simulink model "Copy_2_of_Constant_vel"  (R2024b)
settings: Solver=FixedStepAuto  StartTime=0.0  StopTime=10  FixedStep=0.001  RelTol=1e-3
values from neighbouring files (symbols this model uses):
  marker_data = [marker_data, [20;80;0.5]]    [setup.m]
undefined symbols (not defined in the file or in its folder): r_a, r_b, r_c
libraries: simulink x5, aerolibutil x1, shared6dof x1, aerolibanim x1, aerolibnav x1
(part 2 of 2)

== matlab function Copy_2_of_Constant_vel/MATLAB Function ==
  settings: updateMethod=DISCRETE
  data: z_full input; x_hat_2 output; marker_data parameter; P_hat_2 output
function [x_hat_2, P_hat_2] = fcn(z_full, marker_data)

persistent x_hat_2_prior P_hat_2_prior

dt = 1e-3;

if isempty(x_hat_2_prior)
    x_hat_2_prior = zeros(21,1);
    x_hat_2_prior(1:3) = [0.01 -0.02 0.01];
    x_hat_2_prior(4:6) = [0.01 -0.02 0.11];
    x_hat_2_prior(7:9) = [0 0 0];
    P_hat_2_prior = kron(diag([1e-4 1e-4 1e-12 1e-4 1e-6 1e-6 1e-6]),eye(3));
    x_hat_2_prior(10:12) = [-0.002 0.001 -0.001];
    x_hat_2_prior(13:15) = [0.012 0.022 0.032];
    x_hat_2_prior(16:18) = [0.012 0.022 0.032];
    
end

Q = 0*eye(21);
R = kron(diag([1e-10 1e-14 1e-6 1e-6 1e-6 1e-6]),eye(3));

[r1, r2, r3] = deal(x_hat_2_prior(1), x_hat_2_prior(2), x_hat_2_prior(3));
[r_dot1, r_dot2, r_dot3] = deal(x_hat_2_prior(4), x_hat_2_prior(5), x_hat_2_prior(6));
[r_dot_dot1, r_dot_dot2, r_dot_dot3] = deal(x_hat_2_prior(7), x_hat_2_prior(8), x_hat_2_prior(9));
[eulers1, eulers2, eulers3] = deal(x_hat_2_prior(10), x_hat_2_prior(11), x_hat_2_prior(12));
[eulers_dot1, eulers_dot2, eulers_dot3] = deal(x_hat_2_prior(13), x_hat_2_prior(14), x_hat_2_prior(15));
[omega1, omega2, omega3] = deal(x_hat_2_prior(16), x_hat_2_prior(17), x_hat_2_prior(18));
[omega_dot1, omega_dot2, omega_dot3] = deal(x_hat_2_prior(19), x_hat_2_prior(20), x_hat_2_prior(21));

%Predict
x_hat_1 = [r1+dt.*r_dot1+(dt.^2.*r_dot_dot1)./2.0;
            r2+dt.*r_dot2+(dt.^2.*r_dot_dot2)./2.0;
            r3+dt.*r_dot3+(dt.^2.*r_dot_dot3)./2.0;
            r_dot1+dt.*r_dot_dot1;
            r_dot2+dt.*r_dot_dot2;
            r_dot3+dt.*r_dot_dot3;
            r_dot_dot1;
            r_dot_dot2;
            r_dot_dot3;
            eulers1+dt.*eulers_dot1;
            eulers2+dt.*eulers_dot2;
            eulers3+dt.*eulers_dot3;
            eulers_dot1+dt.*(omega_dot1+omega2.*(eulers_dot1.*cos(eulers1).*tan(eulers2)+eulers_dot2.*1.0./cos(eulers2).^2.*sin(eulers1))-omega3.*(eulers_dot1.*sin(eulers1).*tan(eulers2)-eulers_dot2.*cos(eulers1).*1.0./cos(eulers2).^2)+omega_dot3.*cos(eulers1).*tan(eulers2)+omega_dot2.*sin(eulers1).*tan(eulers2));
            eulers_dot2-dt.*(-omega_dot2.*cos(eulers1)+omega_dot3.*sin(eulers1)+eulers_dot1.*omega2.*sin(eulers1)+eulers_dot1.*omega3.*cos(eulers1));
            eulers_dot3+dt.*(omega2.*((eulers_dot1.*cos(eulers1))./cos(eulers2)+(eulers_dot2.*sin(eulers1).*tan(eulers2))./cos(eulers2))-omega3.*((eulers_dot1.*sin(eulers1))./cos(eulers2)-(eulers_dot2.*cos(eulers1).*tan(eulers2))./cos(eulers2))+(omega_dot3.*cos(eulers1))./cos(eulers2)+(omega_dot2.*sin(eulers1))./cos(eulers2));
            omega1+dt.*omega_dot1;
            omega2+dt.*omega_dot2;
            omega3+dt.*omega_dot3;
            omega_dot1;
            omega_dot2;
            omega_dot3];

F_jacobian = reshape([1.0,0.0,0.0,0.0,0.0,0.0,0.0,0.0,0.0,0.0,0.0,0.0,0.0,0.0,0.0,0.0,0.0,0.0,0.0,0.0,0.0,0.0,1.0,0.0,0.0,0.0,0.0,0.0,0.0,0.0,0.0,0.0,0.0,0.0,0.0,0.0,0.0,0.0,0.0,0.0,0.0,0.0,0.0,0.0,1.0,0.0,0.0,0.0,0.0,0.0,0.0,0.0,0.0,0.0,0.0,0.0,0.0,0.0,0.0,0.0,0.0,0.0,0.0,dt,0.0,0.0,1.0,0.0,0.0,0.0,0.0,0.0,0.0,0.0,0.0,0.0,0.0,0.0,0.0,0.0,0.0,0.0,0.0,0.0,0.0,dt,0.0,0.0,1.0,0.0,0.0,0.0,0.0,0.0,0.0,0.0,0.0,0.0,0.0,0.0,0.0,0.0,0.0,0.0,0.0,0.0,0.0,dt,0.0,0.0,1.0,0.0,0.0,0.0,0.0,0.0,0.0,0.0,0.0,0.0,0.0,0.0,0.0,0.0,0.0,0.0,dt.^2./2.0,0.0,0.0,dt,0.0,0.0,1.0,0.0,0.0,0.0,0.0,0.0,0.0,0.0,0.0,0.0,0.0,0.0,0.0,0.0,0.0,0.0,dt.^2./2.0,0.0,0.0,dt,0.0,0.0,1.0,0.0,0.0,0.0,0.0,0.0,0.0,0.0,0.0,0.0,0.0,0.0,0.0,0.0,0.0,0.0,dt.^2./2.0,0.0,0.0,dt,0.0,0.0,1.0,0.0,0.0,0.0,0.0,0.0,0.0,0.0,0.0,0.0,0.0,0.0,0.0,0.0,0.0,0.0,0.0,0.0,0.0,0.0,0.0,0.0,1.0,0.0,0.0,-dt.*(omega2.*(eulers_dot1.*sin(eulers1).*tan(eulers2)-eulers_dot2.*cos(eulers1).*1.0./cos(eulers2).^2)+omega3.*(eulers_dot1.*cos(eulers1).*tan(eulers2)+eulers_dot2.*1.0./cos(eulers2).^2.*sin(eulers1))-omega_dot2.*cos(eulers1).*tan(eulers2)+omega_dot3.*sin(eulers1).*tan(eulers2)),-dt.*(omega_dot3.*cos(eulers1)+omega_dot2.*sin(eulers1)-eulers_dot1.*omega3.*sin(eulers1)+eulers_dot1.*omega2.*cos(eulers1)),-dt.*(omega2.*((eulers_dot1.*sin(eulers1))./cos(eulers2)-(eulers_dot2.*cos(eulers1).*tan(eulers2))./cos(eulers2))+omega3.*((eulers_dot1.*cos(eulers1))./cos(eulers2)+(eulers_dot2.*sin(eulers1).*tan(eulers2))./cos(eulers2))-(omega_dot2.*cos(eulers1))./cos(eulers2)+(omega_dot3.*sin(eulers1))./cos(eulers2)),0.0,0.0,0.0,0.0,0.0,0.0,0.0,0.0,0.0,0.0,0.0,0.0,0.0,0.0,0.0,0.0,1.0,0.0,dt.*(omega2.*(eulers_dot1.*cos(eulers1).*(tan(eulers2).^2+1.0)+eulers_dot2.*1.0./cos(eulers2).^3.*sin(eulers1).*sin(eulers2).*2.0)-omega3.*(eulers_dot1.*sin(eulers1).*(tan(eulers2).^2+1.0)-eulers_dot2.*cos(eulers1).*1.0./cos(eulers2).^3.*sin(eulers2).*2.0)+omega_dot3.*cos(eulers1).*(tan(eulers2).^2+1.0)+omega_dot2.*sin(eulers1).*(tan(eulers2).^2+1.0)),0.0,dt.*(omega3.*((eulers_dot2.*cos(eulers1).*(tan(eulers2).^2+1.0))./cos(eulers2)-eulers_dot1.*1.0./cos(eulers2).^2.*sin(eulers1).*sin(eulers2)+eulers_dot2.*cos(eulers1).*1.0./cos(eulers2).^2.*sin(eulers2).*tan(eulers2))+omega2.*((eulers_dot2.*sin(eulers1).*(tan(eulers2).^2+1.0))./cos(eulers2)+eulers_dot1.*cos(eulers1).*1.0./cos(eulers2).^2.*sin(eulers2)+eulers_dot2.*1.0./cos(eulers2).^2.*sin(eulers1).*sin(eulers2).*tan(eulers2))+omega_dot3.*cos(eulers1).*1.0./cos(eulers2).^2.*sin(eulers2)+omega_dot2.*1.0./cos(eulers2).^2.*sin(eulers1).*sin(eulers2)),0.0,0.0,0.0,0.0,0.0,0.0,0.0,0.0,0.0,0.0,0.0,0.0,0.0,0.0,0.0,0.0,0.0,1.0,0.0,0.0,0.0,0.0,0.0,0.0,0.0,0.0,0.0,0.0,0.0,0.0,0.0,0.0,0.0,0.0,0.0,0.0,dt,0.0,0.0,dt.*(omega2.*cos(eulers1).*tan(eulers2)-omega3.*sin(eulers1).*tan(eulers2))+1.0,-dt.*(omega3.*cos(eulers1)+omega2.*sin(eulers1)),dt.*((omega2.*cos(eulers1))./cos(eulers2)-(omega3.*sin(eulers1))./cos(eulers2)),0.0,0.0,0.0,0.0,0.0,0.0,0.0,0.0,0.0,0.0,0.0,0.0,0.0,0.0,0.0,0.0,dt,0.0,dt.*(omega3.*cos(eulers1).*1.0./cos(eulers2).^2+omega2.*1.0./cos(eulers2).^2.*sin(eulers1)),1.0,dt.*((omega3.*cos(eulers1).*tan(eulers2))./cos(eulers2)+(omega2.*sin(eulers1).*tan(eulers2))./cos(eulers2)),0.0,0.0,0.0,0.0,0.0,0.0,0.0,0.0,0.0,0.0,0.0,0.0,0.0,0.0,0.0,0.0,0.0,dt,0.0,0.0,1.0,0.0,0.0,0.0,0.0,0.0,0.0,0.0,0.0,0.0,0.0,0.0,0.0,0.0,0.0,0.0,0.0,0.0,0.0,0.0,0.0,0.0,1.0,0.0,0.0,0.0,0.0,0.0,0.0,0.0,0.0,0.0,0.0,0.0,0.0,0.0,0.0,0.0,0.0,0.0,dt.*(eulers_dot1.*cos(eulers1).*tan(eulers2)+eulers_dot2.*1.0./cos(eulers2).^2.*sin(eulers1)),-dt.*eulers_dot1.*sin(eulers1),dt.*((eulers_dot1.*cos(eulers1))./cos(eulers2)+(eulers_dot2.*sin(eulers1).*tan(eulers2))./cos(eulers2)),0.0,1.0,0.0,0.0,0.0,0.0,0.0,0.0,0.0,0.0,0.0,0.0,0.0,0.0,0.0,0.0,0.0,0.0,-dt.*(eulers_dot1.*sin(eulers1).*tan(eulers2)-eulers_dot2.*cos(eulers1).*1.0./cos(eulers2).^2),-dt.*eulers_dot1.*cos(eulers1),-dt.*((eulers_dot1.*sin(eulers1))./cos(eulers2)-(eulers_dot2.*cos(eulers1).*tan(eulers2))./cos(eulers2)),0.0,0.0,1.0,0.0,0.0,0.0,0.0,0.0,0.0,0.0,0.0,0.0,0.0,0.0,0.0,0.0,0.0,0.0,dt,0.0,0.0,dt,0.0,0.0,1.0,0.0,0.0,0.0,0.0,0.0,0.0,0.0,0.0,0.0,0.0,0.0,0.0,0.0,0.0,dt.*sin(eulers1).*tan(eulers2),dt.*cos(eulers1),(dt.*sin(eulers1))./cos(eulers2),0.0,dt,0.0,0.0,1.0,0.0,0.0,0.0,0.0,0.0,0.0,0.0,0.0,0.0,0.0,0.0,0.0,0.0,dt.*cos(eulers1).*tan(eulers2),-dt.*sin(eulers1),(dt.*cos(eulers1))./cos(eulers2),0.0,0.0,dt,0.0,0.0,1.0],[21,21]);
P_hat_1 = F_jacobian*P_hat_2_prior*F_jacobian' + Q;

%Update
%sensor_indicies = sensor_vec==1;
%num_sensors = length(sensor_indicies);
num_sensors = 21;

rho_prediction = zeros(12,1);

H_jacobian_rho = zeros(12,21);
for i=0:3
    marker1 = marker_data(1,i+1);
    marker2 = marker_data(2,i+1);
    marker3 = marker_data(3,i+1);
    rho_prediction(1+(3*i):3+(3*i)) = [1.0./sqrt((marker1-r1).^2+(marker2-r2).^2+(marker3-r3).^2).*(-sin(eulers2).*(marker3-r3)+cos(eulers2).*cos(eulers3).*(marker1-r1)+cos(eulers2).*sin(eulers3).*(marker2-r2));
        1.0./sqrt((marker1-r1).^2+(marker2-r2).^2+(marker3-r3).^2).*(-(cos(eulers1).*sin(eulers3)-cos(eulers3).*sin(eulers1).*sin(eulers2)).*(marker1-r1)+(cos(eulers1).*cos(eulers3)+sin(eulers1).*sin(eulers2).*sin(eulers3)).*(marker2-r2)+cos(eulers2).*sin(eulers1).*(marker3-r3));
        1.0./sqrt((marker1-r1).^2+(marker2-r2).^2+(marker3-r3).^2).*((sin(eulers1).*sin(eulers3)+cos(eulers1).*cos(eulers3).*sin(eulers2)).*(marker1-r1)-(cos(eulers3).*sin(eulers1)-cos(eulers1).*sin(eulers2).*sin(eulers3)).*(marker2-r2)+cos(eulers1).*cos(eulers2).*(marker3-r3))];
    H_jacobian_rho(1+(3*i):3+(3*i),:) = reshape([((marker1.*2.0-r1.*2.0).*1.0./((marker1-r1).^2+(marker2-r2).^2+(marker3-r3).^2).^(3.0./2.0).*(-sin(eulers2).*(marker3-r3)+cos(eulers2).*cos(eulers3).*(marker1-r1)+cos(eulers2).*sin(eulers3).*(marker2-r2)))./2.0-cos(eulers2).*cos(eulers3).*1.0./sqrt((marker1-r1).^2+(marker2-r2).^2+(marker3-r3).^2),(cos(eulers1).*sin(eulers3)-cos(eulers3).*sin(eulers1).*sin(eulers2)).*1.0./sqrt((marker1-r1).^2+(marker2-r2).^2+(marker3-r3).^2)+((marker1.*2.0-r1.*2.0).*1.0./((marker1-r1).^2+(marker2-r2).^2+(marker3-r3).^2).^(3.0./2.0).*(-(cos(eulers1).*sin(eulers3)-cos(eulers3).*sin(eulers1).*sin(eulers2)).*(marker1-r1)+(cos(eulers1).*cos(eulers3)+sin(eulers1).*sin(eulers2).*sin(eulers3)).*(marker2-r2)+cos(eulers2).*sin(eulers1).*(marker3-r3)))./2.0,-(sin(eulers1).*sin(eulers3)+cos(eulers1).*cos(eulers3).*sin(eulers2)).*1.0./sqrt((marker1-r1).^2+(marker2-r2).^2+(marker3-r3).^2)+((marker1.*2.0-r1.*2.0).*1.0./((marker1-r1).^2+(marker2-r2).^2+(marker3-r3).^2).^(3.0./2.0).*((sin(eulers1).*sin(eulers3)+cos(eulers1).*cos(eulers3).*sin(eulers2)).*(marker1-r1)-(cos(eulers3).*sin(eulers1)-cos(eulers1).*sin(eulers2).*sin(eulers3)).*(marker2-r2)+cos(eulers1).*cos(eulers2).*(marker3-r3)))./2.0,((marker2.*2.0-r2.*2.0).*1.0./((marker1-r1).^2+(marker2-r2).^2+(marker3-r3).^2).^(3.0./2.0).*(-sin(eulers2).*(marker3-r3)+cos(eulers2).*cos(eulers3).*(marker1-r1)+cos(eulers2).*sin(eulers3).*(marker2-r2)))./2.0-cos(eulers2).*sin(eulers3).*1.0./sqrt((marker1-r1).^2+(marker2-r2).^2+(marker3-r3).^2),-(cos(eulers1).*cos(eulers3)+sin(eulers1).*sin(eulers2).*sin(eulers3)).*1.0./sqrt((marker1-r1).^2+(marker2-r2).^2+(marker3-r3).^2)+((marker2.*2.0-r2.*2.0).*1.0./((marker1-r1).^2+(marker2-r2).^2+(marker3-r3).^2).^(3.0./2.0).*(-(cos(eulers1).*sin(eulers3)-cos(eulers3).*sin(eulers1).*sin(eulers2)).*(marker1-r1)+(cos(eulers1).*cos(eulers3)+sin(eulers1).*sin(eulers2).*sin(eulers3)).*(marker2-r2)+cos(eulers2).*sin(eulers1).*(marker3-r3)))./2.0,(cos(eulers3).*sin(eulers1)-cos(eulers1).*sin(eulers2).*sin(eulers3)).*1.0./sqrt((marker1-r1).^2+(marker2-r2).^2+(marker3-r3).^2)+((marker2.*2.0-r2.*2.0).*1.0./((marker1-r1).^2+(marker2-r2).^2+(marker3-r3).^2).^(3.0./2.0).*((sin(eulers1).*sin(eulers3)+cos(eulers1).*cos(eulers3).*sin(eulers2)).*(marker1-r1)-(cos(eulers3).*sin(eulers1)-cos(eulers1).*sin(eulers2).*sin(eulers3)).*(marker2-r2)+cos(eulers1).*cos(eulers2).*(marker3-r3)))./2.0,sin(eulers2).*1.0./sqrt((marker1-r1).^2+(marker2-r2).^2+(marker3-r3).^2)+((marker3.*2.0-r3.*2.0).*1.0./((marker1-r1).^2+(marker2-r2).^2+(marker3-r3).^2).^(3.0./2.0).*(-sin(eulers2).*(marker3-r3)+cos(eulers2).*cos(eulers3).*(marker1-r1)+cos(eulers2).*sin(eulers3).*(marker2-r2)))./2.0,((marker3.*2.0-r3.*2.0).*1.0./((marker1-r1).^2+(marker2-r2).^2+(marker3-r3).^2).^(3.0./2.0).*(-(cos(eulers1).*sin(eulers3)-cos(eulers3).*sin(eulers1).*sin(eulers2)).*(marker1-r1)+(cos(eulers1).*cos(eulers3)+sin(eulers1).*sin(eulers2).*sin(eulers3)).*(marker2-r2)+cos(eulers2).*sin(eulers1).*(marker3-r3)))./2.0-cos(eulers2).*sin(eulers1).*1.0./sqrt((marker1-r1).^2+(marker2-r2).^2+(marker3-r3).^2),((marker3.*2.0-r3.*2.0).*1.0./((marker1-r1).^2+(marker2-r2).^2+(marker3-r3).^2).^(3.0./2.0).*((sin(eulers1).*sin(eulers3)+cos(eulers1).*cos(eulers3).*sin(eulers2)).*(marker1-r1)-(cos(eulers3).*sin(eulers1)-cos(eulers1).*sin(eulers2).*sin(eulers3)).*(marker2-r2)+cos(eulers1).*cos(eulers2).*(marker3-r3)))./2.0-cos(eulers1).*cos(eulers2).*1.0./sqrt((marker1-r1).^2+(marker2-r2).^2+(marker3-r3).^2),0.0,0.0,0.0,0.0,0.0,0.0,0.0,0.0,0.0,0.0,0.0,0.0,0.0,0.0,0.0,0.0,0.0,0.0,0.0,1.0./sqrt((marker1-r1).^2+(marker2-r2).^2+(marker3-r3).^2).*((sin(eulers1).*sin(eulers3)+cos(eulers1).*cos(eulers3).*sin(eulers2)).*(marker1-r1)-(cos(eulers3).*sin(eulers1)-cos(eulers1).*sin(eulers2).*sin(eulers3)).*(marker2-r2)+cos(eulers1).*cos(eulers2).*(marker3-r3)),-1.0./sqrt((marker1-r1).^2+(marker2-r2).^2+(marker3-r3).^2).*(-(cos(eulers1).*sin(eulers3)-cos(eulers3).*sin(eulers1).*sin(eulers2)).*(marker1-r1)+(cos(eulers1).*cos(eulers3)+sin(eulers1).*sin(eulers2).*sin(eulers3)).*(marker2-r2)+cos(eulers2).*sin(eulers1).*(marker3-r3)),-1.0./sqrt((marker1-r1).^2+(marker2-r2).^2+(marker3-r3).^2).*(cos(eulers2).*(marker3-r3)+cos(eulers3).*sin(eulers2).*(marker1-r1)+sin(eulers2).*sin(eulers3).*(marker2-r2)),1.0./sqrt((marker1-r1).^2+(marker2-r2).^2+(marker3-r3).^2).*(-sin(eulers1).*sin(eulers2).*(marker3-r3)+cos(eulers2).*cos(eulers3).*sin(eulers1).*(marker1-r1)+cos(eulers2).*sin(eulers1).*sin(eulers3).*(marker2-r2)),1.0./sqrt((marker1-r1).^2+(marker2-r2).^2+(marker3-r3).^2).*(-cos(eulers1).*sin(eulers2).*(marker3-r3)+cos(eulers1).*cos(eulers2).*cos(eulers3).*(marker1-r1)+cos(eulers1).*cos(eulers2).*sin(eulers3).*(marker2-r2)),(cos(eulers2).*cos(eulers3).*(marker2-r2)-cos(eulers2).*sin(eulers3).*(marker1-r1)).*1.0./sqrt((marker1-r1).^2+(marker2-r2).^2+(marker3-r3).^2),-((cos(eulers1).*cos(eulers3)+sin(eulers1).*sin(eulers2).*sin(eulers3)).*(marker1-r1)+(cos(eulers1).*sin(eulers3)-cos(eulers3).*sin(eulers1).*sin(eulers2)).*(marker2-r2)).*1.0./sqrt((marker1-r1).^2+(marker2-r2).^2+(marker3-r3).^2),((cos(eulers3).*sin(eulers1)-cos(eulers1).*sin(eulers2).*sin(eulers3)).*(marker1-r1)+(sin(eulers1).*sin(eulers3)+cos(eulers1).*cos(eulers3).*sin(eulers2)).*(marker2-r2)).*1.0./sqrt((marker1-r1).^2+(marker2-r2).^2+(marker3-r3).^2),0.0,0.0,0.0,0.0,0.0,0.0,0.0,0.0,0.0,0.0,0.0,0.0,0.0,0.0,0.0,0.0,0.0,0.0,0.0,0.0,0.0,0.0,0.0,0.0,0.0,0.0,0.0],[3,21]);
    i = i+1;
end
omega_prediction = [omega1; omega2; omega3];
accel_prediction = [r_dot_dot1; r_dot_dot2; r_dot_dot3];

H_jacobian_accel = reshape([0.0,0.0,0.0,0.0,0.0,0.0,0.0,0.0,0.0,0.0,0.0,0.0,0.0,0.0,0.0,0.0,0.0,0.0,cos(eulers2).*cos(eulers3),-cos(eulers1).*sin(eulers3)+cos(eulers3).*sin(eulers1).*sin(eulers2),sin(eulers1).*sin(eulers3)+cos(eulers1).*cos(eulers3).*sin(eulers2),cos(eulers2).*sin(eulers3),cos(eulers1).*cos(eulers3)+sin(eulers1).*sin(eulers2).*sin(eulers3),-cos(eulers3).*sin(eulers1)+cos(eulers1).*sin(eulers2).*sin(eulers3),-sin(eulers2),cos(eulers2).*sin(eulers1),cos(eulers1).*cos(eulers2),0.0,r_dot_dot1.*(sin(eulers1).*sin(eulers3)+cos(eulers1).*cos(eulers3).*sin(eulers2))-r_dot_dot2.*(cos(eulers3).*sin(eulers1)-cos(eulers1).*sin(eulers2).*sin(eulers3))+r_dot_dot3.*cos(eulers1).*cos(eulers2),r_dot_dot1.*(cos(eulers1).*sin(eulers3)-cos(eulers3).*sin(eulers1).*sin(eulers2))-r_dot_dot2.*(cos(eulers1).*cos(eulers3)+sin(eulers1).*sin(eulers2).*sin(eulers3))-r_dot_dot3.*cos(eulers2).*sin(eulers1),-r_dot_dot3.*cos(eulers2)-r_dot_dot1.*cos(eulers3).*sin(eulers2)-r_dot_dot2.*sin(eulers2).*sin(eulers3),-r_dot_dot3.*sin(eulers1).*sin(eulers2)+r_dot_dot1.*cos(eulers2).*cos(eulers3).*sin(eulers1)+r_dot_dot2.*cos(eulers2).*sin(eulers1).*sin(eulers3),-r_dot_dot3.*cos(eulers1).*sin(eulers2)+r_dot_dot1.*cos(eulers1).*cos(eulers2).*cos(eulers3)+r_dot_dot2.*cos(eulers1).*cos(eulers2).*sin(eulers3),r_dot_dot2.*cos(eulers2).*cos(eulers3)-r_dot_dot1.*cos(eulers2).*sin(eulers3),-r_dot_dot1.*(cos(eulers1).*cos(eulers3)+sin(eulers1).*sin(eulers2).*sin(eulers3))-r_dot_dot2.*(cos(eulers1).*sin(eulers3)-cos(eulers3).*sin(eulers1).*sin(eulers2)),r_dot_dot1.*(cos(eulers3).*sin(eulers1)-cos(eulers1).*sin(eulers2).*sin(eulers3))+r_dot_dot2.*(sin(eulers1).*sin(eulers3)+cos(eulers1).*cos(eulers3).*sin(eulers2)),0.0,0.0,0.0,0.0,0.0,0.0,0.0,0.0,0.0,0.0,0.0,0.0,0.0,0.0,0.0,0.0,0.0,0.0,0.0,0.0,0.0,0.0,0.0,0.0,0.0,0.0,0.0],[3,21]);
H_jacobian_omega = [zeros(3,15),eye(3),zeros(3,3)];

prediction = [accel_prediction; omega_prediction; rho_prediction];
H_jacobian = [H_jacobian_accel; H_jacobian_omega; H_jacobian_rho];

y = z_full - prediction;
S = H_jacobian*P_hat_1*H_jacobian' + R;
K = P_hat_1*H_jacobian'*inv(S);
x_hat_2 = x_hat_1 + K*y;
P_hat_2 = (eye(num_sensors) - K*H_jacobian)*P_hat_1;

x_hat_2_prior = x_hat_2;
P_hat_2_prior = P_hat_2;
